simulink model "final"  (R2024b)
settings: Solver=VariableStepAuto  StartTime=0.0  StopTime=10  RelTol=1e-3
libraries: spsSeriesRLCBranchLib x9, spsIGBTDiodeLib x8, spsThyristorLib x8, spsDiodeLib x5, spsVoltageMeasurementLib x5, spsControlledVoltageSourceLib x4, spsIdealSwitchLib x4, simulink x3, spsCurrentMeasurementLib x2, spsThreePhaseParallelRLCBranchLib x1, spsGroundLib x1, spsPVArrayLib x1
settings Model: Creator=BHISMODEV  LastModifiedBy=BHISMODEV

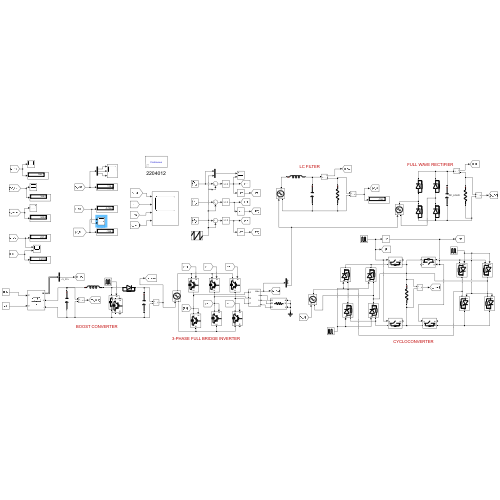
[thumbnail: Simulink's stored preview of the top-level diagram]
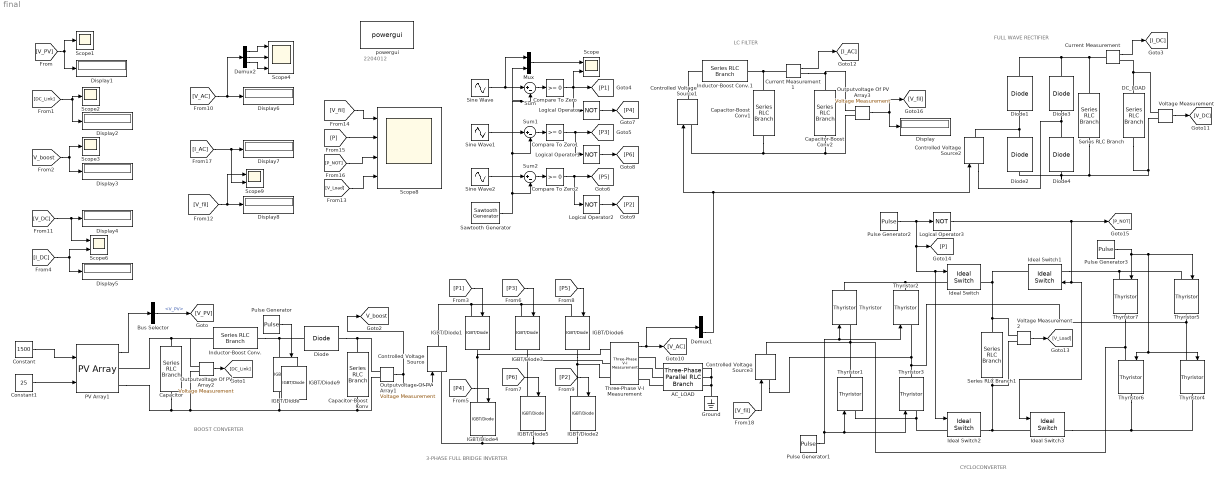
== system final ==
  note: 2204012
  note: FULL WAVE RECTIFIER
  note: BOOST CONVERTER
  note: 3-PHASE FULL BRIDGE INVERTER
  note: CYCLOCONVERTER
  note: LC FILTER
  AC_LOAD : spsThreePhaseParallelRLCBranchLib/Three-Phase Parallel RLC Branch  LConnTagsString=A|B|C  RConnTagsString=A|B|C  BranchType=R  Resistance=1  Inductance=1e-3  Capacitance=1e-6  Measurements=None
  Bus Selector : BusSelector  OutputSignals=V_PV
  Capacitor : spsSeriesRLCBranchLib/Series RLC Branch  LConnTagsString=__new0  RConnTagsString=__new0  BranchType=C  Resistance=1  Inductance=1e-3  SetiL0=off  InitialCurrent=0  Capacitance=0.006  Setx0=off  InitialVoltage=0  Measurements=None
  Capacitor-Boost Conv : spsSeriesRLCBranchLib/Series RLC Branch  LConnTagsString=__new0  RConnTagsString=__new0  BranchType=C  Resistance=1  Inductance=1e-3  SetiL0=off  InitialCurrent=0  Capacitance=0.990  Setx0=off  InitialVoltage=0  Measurements=None
  Capacitor-Boost Conv1 : spsSeriesRLCBranchLib/Series RLC Branch  LConnTagsString=__new0  RConnTagsString=__new0  BranchType=C  Resistance=1  Inductance=1e-3  SetiL0=off  InitialCurrent=0  Capacitance=10e-6  Setx0=off  InitialVoltage=0  Measurements=None
  Capacitor-Boost Conv2 : spsSeriesRLCBranchLib/Series RLC Branch  LConnTagsString=__new0  RConnTagsString=__new0  BranchType=R  Resistance=1000  Inductance=1e-3  SetiL0=off  InitialCurrent=0  Capacitance=0.990  Setx0=off  InitialVoltage=0  Measurements=None
  Compare To Zero : simulink/Logic and Bit Operations/Compare To Zero  relop=>=  OutDataTypeStr=boolean
  Compare To Zero1 : simulink/Logic and Bit Operations/Compare To Zero  relop=>=  OutDataTypeStr=boolean
  Compare To Zero2 : simulink/Logic and Bit Operations/Compare To Zero  relop=>=  OutDataTypeStr=boolean
  Constant : Constant  Value=1500
  Constant1 : Constant  Value=25
  Controlled Voltage Source : spsControlledVoltageSourceLib/Controlled Voltage Source  Initialize=on  Source_Type=DC  Amplitude=100  Phase=0  Frequency=0  Measurements=None
  Controlled Voltage Source1 : spsControlledVoltageSourceLib/Controlled Voltage Source  Initialize=on  Source_Type=AC  Amplitude=0  Phase=0  Frequency=0  Measurements=None
  Controlled Voltage Source2 : spsControlledVoltageSourceLib/Controlled Voltage Source  Initialize=on  Source_Type=AC  Amplitude=0  Phase=0  Frequency=50  Measurements=None
  Controlled Voltage Source3 : spsControlledVoltageSourceLib/Controlled Voltage Source  Initialize=on  Source_Type=AC  Amplitude=0  Phase=0  Frequency=50  Measurements=None
  Current Measurement : spsCurrentMeasurementLib/Current Measurement  PhasorSimulation=off  OutputType=Complex  PSBequivalent=0
  Current Measurement1 : spsCurrentMeasurementLib/Current Measurement  PhasorSimulation=off  OutputType=Complex  PSBequivalent=0
  DC_LOAD : spsSeriesRLCBranchLib/Series RLC Branch  LConnTagsString=__new0  RConnTagsString=__new0  BranchType=R  Resistance=1000  Inductance=0.002  SetiL0=off  InitialCurrent=0  Capacitance=2  Setx0=off  InitialVoltage=0  Measurements=None
  Demux1 : Demux  Outputs=3
  Demux2 : Demux  Outputs=3
  Diode{,1..4} (5 alike) : spsDiodeLib/Diode  Ron=0.001  Lon=0  Vf=0.8  IC=0  UseSnubber=0  Rs=500  Cs=250e-9  Measurements=off
  Display{,1..8} (9 alike) : Display
  Ground : spsGroundLib/Ground  LConnTagsString=a
  IGBT/Diode : spsIGBTDiodeLib/IGBT//Diode  Ron=1e-3  Rs=1e5  Cs=inf  Measurements=on
  IGBT/Diode{1,3..6} (5 alike) : spsIGBTDiodeLib/IGBT//Diode  Ron=1e-3  Rs=1e5  Cs=inf  Measurements=off
  IGBT/Diode2 : spsIGBTDiodeLib/IGBT//Diode  Ron=1e-3  Rs=1e5  Cs=inf  Measurements=on
  IGBT/Diode9 : spsIGBTDiodeLib/IGBT//Diode  Ron=1e-3  Rs=1e5  Cs=inf  Measurements=on
  Ideal Switch{,1..3} (4 alike) : spsIdealSwitchLib/Ideal Switch  Ron=0.001  Lon=0  IC=0  Rs=1e5  Cs=inf  Measurements=on
  Inductor-Boost Conv. : spsSeriesRLCBranchLib/Series RLC Branch  LConnTagsString=__new0  RConnTagsString=__new0  BranchType=L  Resistance=1  Inductance=0.08  SetiL0=off  InitialCurrent=0  Capacitance=1e-6  Setx0=off  InitialVoltage=0  Measurements=None
  Inductor-Boost Conv.1 : spsSeriesRLCBranchLib/Series RLC Branch  LConnTagsString=__new0  RConnTagsString=__new0  BranchType=L  Resistance=1  Inductance=0.05  SetiL0=off  InitialCurrent=0  Capacitance=1e-6  Setx0=off  InitialVoltage=0  Measurements=None
  Logical Operator{,1..3} (4 alike) : Logic  Operator=NOT  AllPortsSameDT=off  OutDataTypeStr=boolean
  Mux : Mux  Inputs=2
  Outputvoltage Of PV Array1 : spsVoltageMeasurementLib/Voltage Measurement  PhasorSimulation=off  OutputType=Complex  PSBequivalent=0
  Outputvoltage Of PV Array2 : spsVoltageMeasurementLib/Voltage Measurement  PhasorSimulation=off  OutputType=Complex  PSBequivalent=0
  Outputvoltage Of PV Array3 : spsVoltageMeasurementLib/Voltage Measurement  PhasorSimulation=off  OutputType=Complex  PSBequivalent=0
  PV Array1 : spsPVArrayLib/PV Array  Npar=20  Nser=4.5  PlotType=array @ 1000 W/m2 & specified temperatures  S_vec="[ 1000  500  100 ]"  Temp_C_vec="[ 45 25  ]"  ModuleName=User-defined  PlotWhenSelected=off  Pm=213.15  Ncell=60  Voc=36.3  Isc=7.84  Vm=29  Im=7.35  beta_Voc_pc=-0.36099  alpha_Isc_pc=0.102  beta_Voc=-0.13104  alpha_Isc=0.0079968  IL=7.8654  I0=2.9273e-10  nI=0.98119  Rsh=313.0553  Rs=0.39381  RobustModel=off  RobustCellTemperature=313.3991  BAL=on  Tc=1e-6  Tfilter=5e-5
  Pulse Generator : DiscretePulseGenerator  PulseType=Time based  Period=1/15000  PulseWidth=50
  Pulse Generator1 : DiscretePulseGenerator  PulseType=Time based  Period=0.01  PulseWidth=5
  Pulse Generator2 : DiscretePulseGenerator  PulseType=Time based  Period=0.04  PulseWidth=50
  Pulse Generator3 : DiscretePulseGenerator  PulseType=Time based  Period=0.01  PulseWidth=5
  Sawtooth Generator : spsSawtoothGeneratorLib/Sawtooth Generator  Freq=1e3  Phase=180  Ts=0
  Scope : Scope  NumInputPorts=2
  Scope1 : Scope
  Scope2 : Scope
  Scope3 : Scope
  Scope4 : Scope  NumInputPorts=3
  Scope6 : Scope  NumInputPorts=2
  Scope8 : Scope  NumInputPorts=4
  Scope9 : Scope  NumInputPorts=2
  Series RLC Branch : spsSeriesRLCBranchLib/Series RLC Branch  LConnTagsString=__new0  RConnTagsString=__new0  BranchType=C  Resistance=1  Inductance=1e-3  SetiL0=off  InitialCurrent=0  Capacitance=0.4  Setx0=off  InitialVoltage=0  Measurements=None
  Series RLC Branch1 : spsSeriesRLCBranchLib/Series RLC Branch  LConnTagsString=__new0  RConnTagsString=__new0  BranchType=R  Resistance=1  Inductance=1e-3  SetiL0=off  InitialCurrent=0  Capacitance=1e-6  Setx0=off  InitialVoltage=0  Measurements=None
  Sine Wave : Sin  Frequency=2*pi*50  SampleTime=0
  Sine Wave1 : Sin  Frequency=2*pi*50  Phase=2*pi/3  SampleTime=0
  Sine Wave2 : Sin  Frequency=2*pi*50  Phase=-2*pi/3  SampleTime=0
  Sum : Sum  Inputs=|+-
  Sum1 : Sum  Inputs=|+-
  Sum2 : Sum  Inputs=|+-
  Three-Phase V-I Measurement : spsThreePhaseVIMeasurementLib/Three-Phase V-I Measurement  VoltageMeasurement=phase-to-ground  SetLabelV=off  LabelV=Vabc  Vpu=off  VpuLL=off  CurrentMeasurement=no  SetLabelI=off  LabelI=Iabc  Ipu=off  Pbase=100e6  Vbase=500e3  OutputType=Complex  PhasorSimulation=off  PSBequivalent=0
  Thyristor{,1..7} (8 alike) : spsThyristorLib/Thyristor  Ron=0.001  Lon=0  Vf=0.8  IC=0  Rs=500  Cs=250e-9  Measurements=off
  Voltage Measurement : spsVoltageMeasurementLib/Voltage Measurement  PhasorSimulation=off  OutputType=Complex  PSBequivalent=0
  Voltage Measurement2 : spsVoltageMeasurementLib/Voltage Measurement  PhasorSimulation=off  OutputType=Complex  PSBequivalent=0
  powergui : spspowerguiLib/powergui  Priority=1  SimulationMode=Continuous  SampleTime=50e-6  frequency=60  Iterations=50  frequencyindice=0  Pbase=100e6  ErrMax=1e-4  UnitsV=kV  UnitsW=MW  buscounter=0  FunctionMessages=off  echomessages=off  EnableUseOfTLC=off  CurrentSourceSwitches=off  DisableSnubberDevices=off  DisableRonSwitches=off  DisableVfSwitches=off  DisplayEquations=off  AutomaticDiscreteSolvers=off  SolverType=Tustin/Backward Euler (TBE)  Interpol=off  ExternalGateDelay=off  methode=off  Ts=100  x0status=blocks  SPID=on  SwTol=0  HookPort=off  NonlinearTolerance=1e-4  nMaxIteration=100  ContinueOnMaxIteration=off  RestoreLinks=warning  ResistiveCurrentMeasurement=off  Frange=[0:2:500]  Ylog=off  Xlog=on  ShowGrid=off  save=off  variable=ZData  structure=0  ZoomFFT=off  StartTime=0.0  cycles=1  DisplayStyle=1  fundamental=60  FreqAxis=off  MaxFrequency=1000  frequencyindicesteady=1  RmsSteady=1  display=off
  tag scope: V_boost=global
  wires:
  Constant1/1 -> PV Array1/2
  Pulse Generator/1 -> IGBT/Diode/1
  Constant/1 -> PV Array1/1
  PV Array1/1 -> Bus Selector/1
  Bus Selector/1 -> [V_PV]  "<V_PV>"
  [V_PV] -> Display1/1, Scope1/1
  Outputvoltage Of PV Array2/1 -> [DC_Link]
  [DC_Link] -> Display2/1, Scope2/1
  Outputvoltage Of PV Array1/1 -> [V_boost], Controlled Voltage Source/1
  [V_boost] -> Display3/1, Scope3/1
  [P2] -> IGBT/Diode2/1
  Sine Wave2/1 -> Sum2/1
  Sine Wave/1 -> Sum/1, Mux/1
  Compare To Zero2/1 -> [P5], Logical Operator2/1
  Sum/1 -> Compare To Zero/1
  Mux/1 -> Scope/1
  Sum2/1 -> Compare To Zero2/1
  Sum1/1 -> Compare To Zero1/1
  Logical Operator/1 -> [P4]
  Logical Operator2/1 -> [P2]
  Sawtooth Generator/1 -> Sum2/2, Sum1/2, Mux/2, Sum/2
  [P5] -> IGBT/Diode6/1
  [P4] -> IGBT/Diode4/1
  Compare To Zero/1 -> Scope/2, [P1], Logical Operator/1
  Sine Wave1/1 -> Sum1/1
  [P3] -> IGBT/Diode3/1
  Logical Operator1/1 -> [P6]
  Compare To Zero1/1 -> [P3], Logical Operator1/1
  [P1] -> IGBT/Diode1/1
  [P6] -> IGBT/Diode5/1
  Current Measurement/1 -> [I_DC]
  Voltage Measurement/1 -> [V_DC]
  [V_DC] -> Scope6/1, Display4/1
  [I_DC] -> Scope6/2, Display5/1
  Pulse Generator1/1 -> Thyristor2/1, Thyristor/1, Thyristor1/1, Thyristor3/1
  Pulse Generator2/1 -> Ideal Switch2/1, Ideal Switch/1, [P], Logical Operator3/1
  Voltage Measurement2/1 -> [V_Load]
  Pulse Generator3/1 -> Thyristor6/1, Thyristor4/1, Thyristor5/1, Thyristor7/1
  Logical Operator3/1 -> Ideal Switch3/1, Ideal Switch1/1, [P_NOT]
  [P] -> Scope8/2
  [V_fil] -> Scope8/1
  [P_NOT] -> Scope8/3
  [V_Load] -> Scope8/4
  Three-Phase V-I Measurement/1 -> Demux1/1, [V_AC]
  Demux1/3 -> Controlled Voltage Source2/1, Controlled Voltage Source1/1
  [V_fil] -> Controlled Voltage Source3/1
  Outputvoltage Of PV Array3/1 -> [V_fil], Display/1
  [V_AC] -> Display6/1, Demux2/1
  Current Measurement1/1 -> [I_AC]
  [I_AC] -> Scope9/2, Display7/1
  [V_fil] -> Display8/1, Scope9/1
  Demux2/1 -> Scope4/1
  Demux2/2 -> Scope4/2
  Demux2/3 -> Scope4/3
  connections:
  Capacitor/LConn1 -- Inductor-Boost Conv./LConn1 -- Outputvoltage Of PV Array2/LConn1 -- PV Array1/RConn1
  Inductor-Boost Conv./RConn1 -- Diode/LConn1 -- IGBT/Diode/LConn1
  IGBT/Diode6/LConn1 -- IGBT/Diode1/LConn1 -- Controlled Voltage Source/RConn1 -- IGBT/Diode3/LConn1
  Three-Phase V-I Measurement/LConn2 -- IGBT/Diode3/RConn1 -- IGBT/Diode5/LConn1
  IGBT/Diode1/RConn1 -- Three-Phase V-I Measurement/LConn1 -- IGBT/Diode4/LConn1
  IGBT/Diode6/RConn1 -- Three-Phase V-I Measurement/LConn3 -- IGBT/Diode2/LConn1
  AC_LOAD/RConn2 -- AC_LOAD/RConn3 -- Ground/LConn1 -- AC_LOAD/RConn1
  AC_LOAD/LConn3 -- Three-Phase V-I Measurement/RConn3
  AC_LOAD/LConn2 -- Three-Phase V-I Measurement/RConn2
  AC_LOAD/LConn1 -- Three-Phase V-I Measurement/RConn1
  PV Array1/RConn2 -- Capacitor/RConn1 -- Outputvoltage Of PV Array2/LConn2 -- Outputvoltage Of PV Array1/LConn2 -- Capacitor-Boost Conv/RConn1 -- IGBT/Diode/RConn1
  Diode/RConn1 -- Outputvoltage Of PV Array1/LConn1 -- Capacitor-Boost Conv/LConn1
  IGBT/Diode4/RConn1 -- Controlled Voltage Source/LConn1 -- IGBT/Diode5/RConn1 -- IGBT/Diode2/RConn1
  Capacitor-Boost Conv2/LConn1 -- Outputvoltage Of PV Array3/LConn1 -- Current Measurement1/RConn1
  Capacitor-Boost Conv2/RConn1 -- Outputvoltage Of PV Array3/LConn2 -- Controlled Voltage Source1/LConn1 -- Capacitor-Boost Conv1/RConn1
  Diode3/LConn1 -- Controlled Voltage Source2/LConn1 -- Diode4/RConn1
  Diode1/RConn1 -- Current Measurement/LConn1 -- Series RLC Branch/LConn1 -- Diode3/RConn1
  Series RLC Branch/RConn1 -- Voltage Measurement/LConn2 -- DC_LOAD/RConn1 -- Diode4/LConn1 -- Diode2/LConn1
  Controlled Voltage Source2/RConn1 -- Diode2/RConn1 -- Diode1/LConn1
  DC_LOAD/LConn1 -- Voltage Measurement/LConn1 -- Current Measurement/RConn1
  Thyristor/RConn1 -- Ideal Switch/LConn1 -- Thyristor2/RConn1
  Series RLC Branch1/RConn1 -- Voltage Measurement2/LConn2 -- Ideal Switch3/LConn1 -- Ideal Switch2/RConn1
  Series RLC Branch1/LConn1 -- Ideal Switch1/RConn1 -- Ideal Switch/RConn1 -- Voltage Measurement2/LConn1
  Thyristor5/RConn1 -- Thyristor4/LConn1 -- Controlled Voltage Source3/LConn1 -- Thyristor2/LConn1 -- Thyristor3/RConn1
  Thyristor3/LConn1 -- Thyristor1/LConn1 -- Ideal Switch2/LConn1
  Thyristor4/RConn1 -- Thyristor6/RConn1 -- Ideal Switch3/RConn1
  Thyristor/LConn1 -- Thyristor1/RConn1 -- Thyristor7/RConn1 -- Thyristor6/LConn1 -- Controlled Voltage Source3/RConn1
  Thyristor5/LConn1 -- Ideal Switch1/LConn1 -- Thyristor7/LConn1
  Controlled Voltage Source1/RConn1 -- Inductor-Boost Conv.1/LConn1
  Capacitor-Boost Conv1/LConn1 -- Current Measurement1/LConn1 -- Inductor-Boost Conv.1/RConn1
